simulink model "simulation_5"  (R2023b)
settings: Solver=VariableStepAuto  StartTime=0.0  StopTime=10.0  RelTol=1e-3
values from neighbouring files (symbols this model uses):
  b = 1    [script_5.m]
  omega = omegaVals(it, jt)    [script_5.m]
  xi = dampingVals(it, jt)    [script_5.m]
settings Model: Creator=igorkrzywda  LastModifiedBy=igorkrzywda

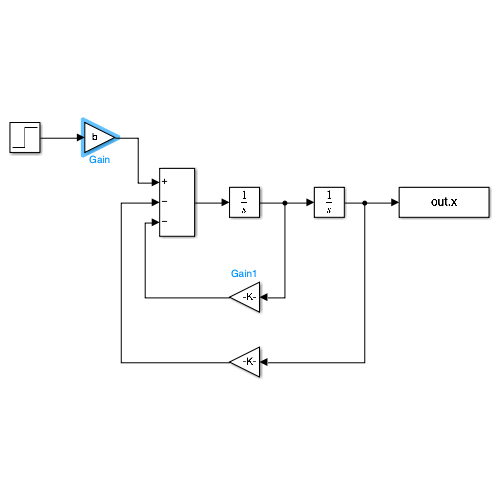
[thumbnail: Simulink's stored preview of the top-level diagram]
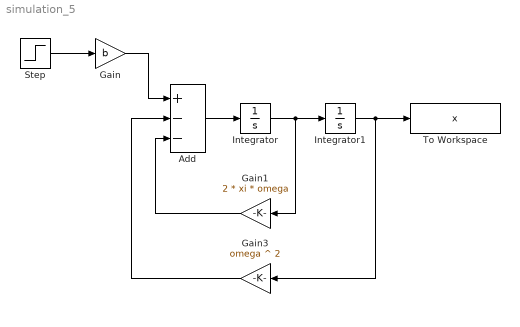
== system simulation_5 ==
  Add : Sum  Inputs=+--
  Gain : Gain  Gain=b
  Gain1 : Gain  Gain=2 * xi * omega
  Gain3 : Gain  Gain=omega ^ 2
  Integrator : Integrator
  Integrator1 : Integrator
  Step : Step  Time=0  SampleTime=0
  To Workspace : ToWorkspace  VariableName=x  SampleTime=-1
  wires:
  Step/1 -> Gain/1
  Gain/1 -> Add/1
  Add/1 -> Integrator/1
  Integrator/1 -> Gain1/1, Integrator1/1
  Integrator1/1 -> To Workspace/1, Gain3/1
  Gain1/1 -> Add/3
  Gain3/1 -> Add/2
